simulink model "drifting_controller_stabilization"  (R2017a)
settings: Solver=FixedStepAuto  StartTime=0.0  StopTime=inf  FixedStep=0.01  RelTol=1e-3
InitFcn:
  | drifting_controller_stabilization_callback
values from neighbouring files (symbols this model uses):
  delta_eqpoint = -20*pi/180    (= -0.349065850399)    [drifting_controller_stabilization_callback.m]
  delta_max = 45*pi/180    (= 0.785398163397)    [drifting_controller_stabilization_callback.m]
  delta_min = -delta_max    (= -0.785398163397)    [drifting_controller_stabilization_callback.m]
  Den_Filter = FilterDTF.Den{1}    [drifting_controller_stabilization_callback.m]
  Fdrag = 1.75    [drifting_controller_stabilization_callback.m]
  Fxr_eqpoint = 3.006    [drifting_controller_stabilization_callback.m]
  Imax = 13    [drifting_controller_stabilization_callback.m]
  K_r_delta = 0.6146    [drifting_controller_stabilization_callback.m]
  K_r_Fxr = 0.8143    [drifting_controller_stabilization_callback.m]
  K_Vx_delta = -0.8304    [drifting_controller_stabilization_callback.m]
  K_Vx_Fxr = 1.2987    [drifting_controller_stabilization_callback.m]
  K_Vy_delta = -0.9889    [drifting_controller_stabilization_callback.m]
  K_Vy_Fxr = -6.6663    [drifting_controller_stabilization_callback.m]
  Kt = 1/340.34    (= 0.00293823823236)    [drifting_controller_stabilization_callback.m]
  Num_Filter = FilterDTF.Num{1}    [drifting_controller_stabilization_callback.m]
  r_eqpoint = 2.31807    [drifting_controller_stabilization_callback.m]
  Rw = 0.049    [drifting_controller_stabilization_callback.m]
  tau = 0.09799    [drifting_controller_stabilization_callback.m]
  Vx_eqpoint = 1.0    (= 1)    [drifting_controller_stabilization_callback.m]
  Vy_eqpoint = -0.7880    (= -0.788)    [drifting_controller_stabilization_callback.m]
undefined symbols (not defined in the file or in its folder): SpeedRef, State, SteerRef
libraries: robotlib x5, aerolibutil x2, sharedtransform x2
settings Model: Creator=bascetta  LastModifiedBy=marco
settings OptimizationCC: ConditionallyExecuteInputs=off  PassReuseOutputArgsAs=Individual arguments  LifeSpan=inf  MaxStackSize=64
settings DebuggingCC: ReadBeforeWriteMsg=EnableAllAsError  WriteAfterWriteMsg=EnableAllAsError  WriteAfterReadMsg=EnableAllAsError  IntegerOverflowMsg=error  ParameterTunabilityLossMsg=error  UniqueDataStoreMsg=error  NonBusSignalsTreatedAsBus=error  SFInvalidInputDataAccessInChartInitDiag=error  SFTransitionOutsideNaturalParentDiag=error  SFUnreachableExecutionPathDiag=error  SFUndirectedBroadcastEventsDiag=error  IntegerSaturationMsg=error
settings HardwareCC: ProdBitPerPointer=32  ProdBitPerSizeT=32  ProdBitPerPtrDiffT=32  ProdLargestAtomicFloat=None  ProdIntDivRoundTo=Undefined  ProdEndianess=Unspecified  ProdWordSize=32  ProdHWDeviceType=Generic->Unspecified (assume 32-bit Generic)
settings SFSimCC: MATLABDynamicMemAlloc=off
settings RTWCC: SystemTargetFile=ert.tlc  HardwareBoard=Robot Operating System (ROS)  TLCOptions="-aInlineSetEventsForThisBaseRateFcn=TLC_FALSE -aSuppressMultiTaskScheduler=TLC_FALSE  -aRateBasedStepFcn=0"  TemplateMakefile=ert_default_tmf  Description=Embedded Coder  GenerateReport=on  Toolchain=Catkin  IncludeHyperlinkInReport=on  LaunchReport=on  TargetLang=C++  GenerateTraceInfo=on  GenerateTraceReport=on  GenerateTraceReportSl=on  GenerateTraceReportSf=on  GenerateTraceReportEml=on
settings CodeAppCC: ForceParamTrailComments=on  IgnoreCustomStorageClasses=off  OperatorAnnotations=on  SimulinkDataObjDesc=on  SFDataObjDesc=on  MATLABFcnDesc=on  InsertBlockDesc=on  MATLABSourceComments=on
settings ERTTargetCC: SupportContinuousTime=on
settings ConfigComp: CovScope=ReferencedModels  CovIncludeTopModel=off

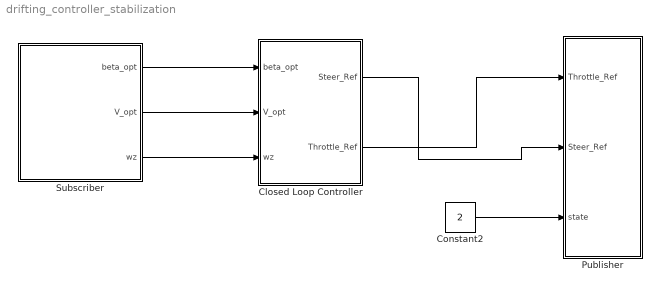
== system drifting_controller_stabilization ==
  Closed Loop Controller : Subsystem
  Constant2 : Constant  Value=2  OutDataTypeStr=uint8
  Publisher : Subsystem
  "Subscriber " : Subsystem
  wires:
  "Subscriber "/1(beta_opt) -> Closed Loop Controller/1(beta_opt)
  "Subscriber "/3(wz) -> Closed Loop Controller/3(wz)
  "Subscriber "/2(V_opt) -> Closed Loop Controller/2(V_opt)
  Closed Loop Controller/2(Throttle_Ref) -> Publisher/1(Throttle_Ref)
  Constant2/1 -> Publisher/3(state)
  Closed Loop Controller/1(Steer_Ref) -> Publisher/2(Steer_Ref)

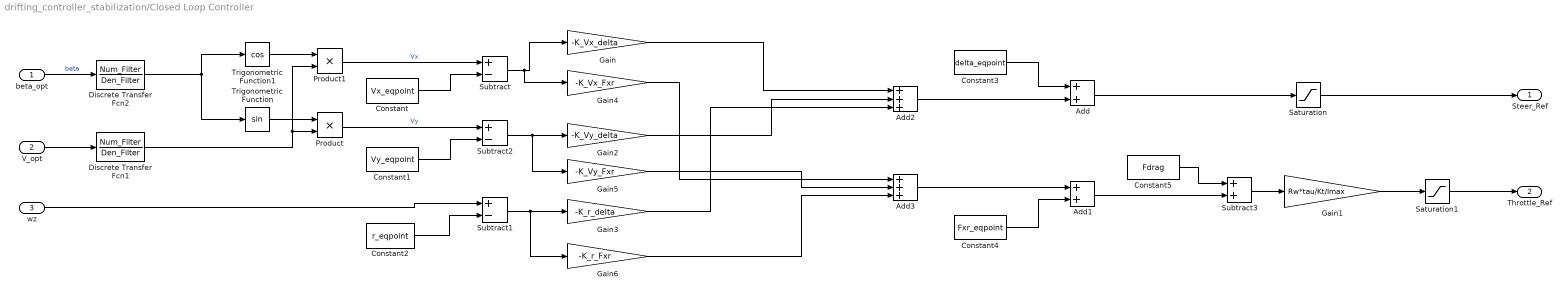
== system drifting_controller_stabilization/Closed Loop Controller ==
  beta_opt : Inport
  V_opt : Inport  Port=2
  wz : Inport  Port=3
  Add : Sum
  Add1 : Sum
  Add2 : Sum  Inputs=+++
  Add3 : Sum  Inputs=+++
  Constant : Constant  Value=Vx_eqpoint
  Constant1 : Constant  Value=Vy_eqpoint
  Constant2 : Constant  Value=r_eqpoint
  Constant3 : Constant  Value=delta_eqpoint
  Constant4 : Constant  Value=Fxr_eqpoint
  Constant5 : Constant  Value=Fdrag
  Discrete Transfer Fcn1 : DiscreteTransferFcn  Numerator=Num_Filter  Denominator=Den_Filter
  Discrete Transfer Fcn2 : DiscreteTransferFcn  Numerator=Num_Filter  Denominator=Den_Filter
  Gain : Gain  Gain=-K_Vx_delta
  Gain1 : Gain  Gain=Rw*tau/Kt/Imax
  Gain2 : Gain  Gain=-K_Vy_delta
  Gain3 : Gain  Gain=-K_r_delta
  Gain4 : Gain  Gain=-K_Vx_Fxr
  Gain5 : Gain  Gain=-K_Vy_Fxr
  Gain6 : Gain  Gain=-K_r_Fxr
  Product : Product
  Product1 : Product
  Saturation : Saturate  UpperLimit=delta_max  LowerLimit=delta_min
  Saturation1 : Saturate  UpperLimit=1  LowerLimit=-1
  Subtract : Sum  Inputs=+-
  Subtract1 : Sum  Inputs=+-
  Subtract2 : Sum  Inputs=+-
  Subtract3 : Sum
  Trigonometric Function : Trigonometry
  Trigonometric Function1 : Trigonometry  Operator=cos
  Steer_Ref : Outport
  Throttle_Ref : Outport  Port=2
  wires:
  beta_opt/1 -> Discrete Transfer Fcn2/1  "beta"
  Trigonometric Function1/1 -> Product1/1
  Trigonometric Function/1 -> Product/1
  Product1/1 -> Subtract/1  "Vx"
  Product/1 -> Subtract2/1  "Vy"
  Constant/1 -> Subtract/2
  Constant1/1 -> Subtract2/2
  Constant2/1 -> Subtract1/2
  Constant3/1 -> Add/1
  Constant4/1 -> Add1/2
  Add1/1 -> Subtract3/2
  Subtract3/1 -> Gain1/1
  Constant5/1 -> Subtract3/1
  Gain1/1 -> Saturation1/1
  Saturation1/1 -> Throttle_Ref/1
  Add/1 -> Saturation/1
  Saturation/1 -> Steer_Ref/1
  Subtract/1 -> Gain4/1, Gain/1
  Subtract2/1 -> Gain5/1, Gain2/1
  Subtract1/1 -> Gain6/1, Gain3/1
  Add2/1 -> Add/2
  Gain/1 -> Add2/1
  Gain2/1 -> Add2/2
  Gain3/1 -> Add2/3
  Add3/1 -> Add1/1
  Gain4/1 -> Add3/1
  Gain6/1 -> Add3/3
  Gain5/1 -> Add3/2
  V_opt/1 -> Discrete Transfer Fcn1/1
  wz/1 -> Subtract1/1
  Discrete Transfer Fcn1/1 -> Product/2, Product1/2
  Discrete Transfer Fcn2/1 -> Trigonometric Function/1, Trigonometric Function1/1

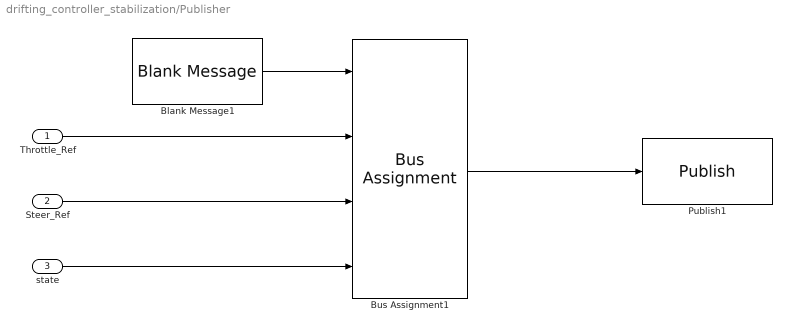
== system drifting_controller_stabilization/Publisher ==
  Throttle_Ref : Inport
  Steer_Ref : Inport  Port=2
  state : Inport  Port=3
  Blank Message1 : robotlib/Blank Message  SourceLibraryInfo=This block requires Robotics System Toolbox  messageType=car_msgs/car_cmd  SampleTime=inf
      settings: SourceProductBaseCode=RO
  Bus Assignment1 : BusAssignment  AssignedSignals=SpeedRef,SteerRef,State
  Publish1 : robotlib/Publish  SourceLibraryInfo=This block requires Robotics System Toolbox  topicSource=Specify your own  topic=/controller_cmd  messageType=car_msgs/car_cmd  messageQueueLength=1
      settings: SourceProductBaseCode=RO
  wires:
  Blank Message1/1 -> Bus Assignment1/1
  Bus Assignment1/1 -> Publish1/1
  Throttle_Ref/1 -> Bus Assignment1/2
  Steer_Ref/1 -> Bus Assignment1/3
  state/1 -> Bus Assignment1/4

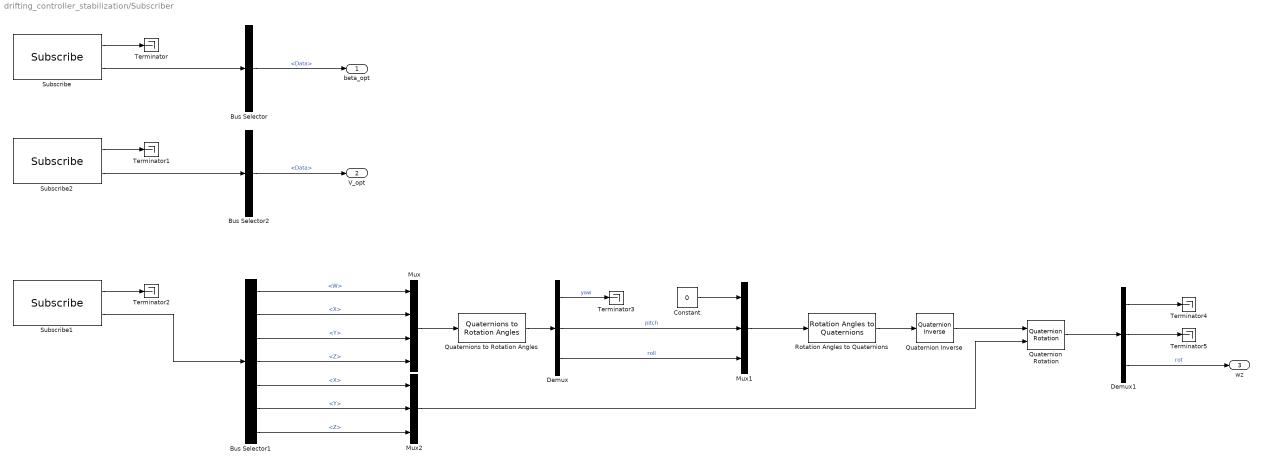
== system drifting_controller_stabilization/Subscriber  ==
  Bus Selector : BusSelector  OutputSignals=Data
  Bus Selector1 : BusSelector  OutputSignals=Orientation.W,Orientation.X,Orientation.Y,Orientation.Z,AngularVelocity.X,AngularVelocity.Y,AngularVelocity.Z
  Bus Selector2 : BusSelector  OutputSignals=Data
  Constant : Constant  Value=0
  Demux : Demux  Outputs=3
  Demux1 : Demux  Outputs=3
  Mux : Mux
  Mux1 : Mux  Inputs=3
  Mux2 : Mux  Inputs=3
  Quaternion Inverse : aerolibutil/Quaternion Inverse
      settings: SourceProductName=Aerospace Blockset
  Quaternion Rotation : aerolibutil/Quaternion Rotation
  Quaternions to Rotation Angles : sharedtransform/Quaternions to Rotation Angles  rotationOrder=ZYX
  Rotation Angles to Quaternions : sharedtransform/Rotation Angles to Quaternions  rotationOrder=ZYX
  Subscribe : robotlib/Subscribe  SourceLibraryInfo=This block requires Robotics System Toolbox  topicSource=Select from ROS network  topic=/state_estimator_opt_beta  messageType=std_msgs/Float64  sampleTime=-1  messageQueueLength=1
      settings: SourceProductBaseCode=RO
  Subscribe1 : robotlib/Subscribe  SourceLibraryInfo=This block requires Robotics System Toolbox  topicSource=Select from ROS network  topic=/imu/data  messageType=sensor_msgs/Imu  sampleTime=-1  messageQueueLength=1
      settings: SourceProductBaseCode=RO
  Subscribe2 : robotlib/Subscribe  SourceLibraryInfo=This block requires Robotics System Toolbox  topicSource=Select from ROS network  topic=/state_estimator_opt_V  messageType=std_msgs/Float64  sampleTime=-1  messageQueueLength=1
      settings: SourceProductBaseCode=RO
  Terminator{,1..5} (6 alike) : Terminator
  beta_opt : Outport
  V_opt : Outport  Port=2
  wz : Outport  Port=3
  wires:
  Subscribe/2 -> Bus Selector/1
  Subscribe2/2 -> Bus Selector2/1
  Bus Selector/1 -> beta_opt/1  "<Data>"
  Bus Selector2/1 -> V_opt/1  "<Data>"
  Subscribe/1 -> Terminator/1
  Subscribe2/1 -> Terminator1/1
  Subscribe1/1 -> Terminator2/1
  Subscribe1/2 -> Bus Selector1/1
  Mux/1 -> Quaternions to Rotation Angles/1
  Bus Selector1/4 -> Mux/4  "<Z>"
  Bus Selector1/3 -> Mux/3  "<Y>"
  Bus Selector1/2 -> Mux/2  "<X>"
  Bus Selector1/1 -> Mux/1  "<W>"
  Quaternions to Rotation Angles/1 -> Demux/1
  Demux/1 -> Terminator3/1  "yaw"
  Constant/1 -> Mux1/1
  Demux/2 -> Mux1/2  "pitch"
  Demux/3 -> Mux1/3  "roll"
  Mux1/1 -> Rotation Angles to Quaternions/1
  Rotation Angles to Quaternions/1 -> Quaternion Inverse/1
  Bus Selector1/6 -> Mux2/2  "<Y>"
  Bus Selector1/5 -> Mux2/1  "<X>"
  Bus Selector1/7 -> Mux2/3  "<Z>"
  Mux2/1 -> Quaternion Rotation/2
  Quaternion Rotation/1 -> Demux1/1
  Quaternion Inverse/1 -> Quaternion Rotation/1
  Demux1/3 -> wz/1  "rot"
  Demux1/1 -> Terminator4/1
  Demux1/2 -> Terminator5/1
